simulink model "Arduino_model"  (R2021a)
settings: Solver=FixedStepAuto  StartTime=0.0  StopTime=inf  FixedStep=0.01  RelTol=1e-3  EnableMultiTasking=on
libraries: arduinolib x4, pid_lib x1, dspsigops x1, svdutilitieslib x1
settings Model: SimulationMode=external  SILPILModeSetting=veronly  ExtModeTrigDuration=2  Creator=s269684  LastModifiedBy=root
settings OptimizationCC: EnhancedBackFolding=on  PassReuseOutputArgsAs=Individual arguments  ZeroExternalMemoryAtStartup=off  ZeroInternalMemoryAtStartup=off  MaxStackSize=64  OptimizeBlockOrder=speed  DifferentSizesBufferReuse=on  OptimizationCustomize=off  EfficientTunableParamExpr=on
settings DebuggingCC: ParameterTunabilityLossMsg=error
settings HardwareCC: ProdBitPerInt=16  ProdBitPerPointer=16  ProdBitPerSizeT=16  ProdBitPerPtrDiffT=16  ProdLargestAtomicFloat=None  ProdWordSize=8  ProdHWDeviceType=Atmel->AVR  UseEmbeddedCoderFeatures=off
settings SFSimCC: MATLABDynamicMemAlloc=off
settings RTWCC: SystemTargetFile=ert.tlc  HardwareBoard=Arduino Uno  TemplateMakefile=ert_default_tmf  Toolchain=Arduino AVR  BuildConfiguration=Faster Runs
settings CodeAppCC: ForceParamTrailComments=on  IgnoreCustomStorageClasses=off  OperatorAnnotations=on  SimulinkDataObjDesc=on  SFDataObjDesc=on  InsertBlockDesc=on
settings ERTTargetCC: SupportContinuousTime=on  SupportNonInlinedSFcns=on  SupportVariableSizeSignals=on  ExtModeStaticAllocSize=250

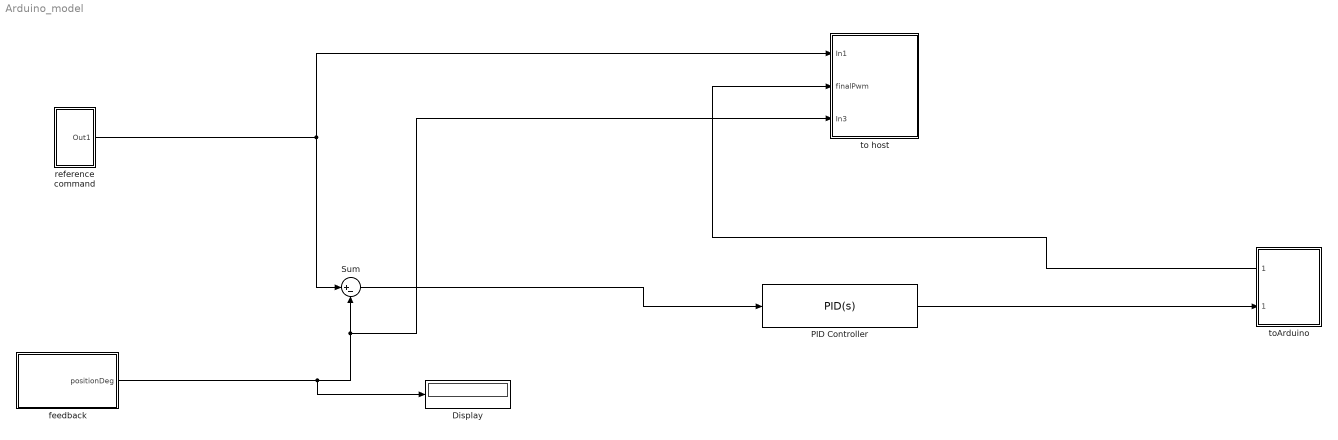
== system Arduino_model ==
  Display : Display
  PID Controller : pid_lib/PID Controller  Controller=PID  Form=Parallel  TimeDomain=Continuous-time  UseExternalTs=off  SampleTime=-1  IntegratorMethod=Forward Euler  FilterMethod=Forward Euler  ControllerParametersSource=internal  P=0.1  I=0  D=0  UseFilter=on  N=100  TunerSelectOption=Transfer Function Based (PID Tuner App)  InitialConditionSource=internal  InitialConditionForIntegrator=0  InitialConditionForFilter=0  DifferentiatorICPrevScaledInput=0  ExternalReset=none  TrackingMode=off  Kt=1  LimitOutput=off  SatLimitsSource=internal  UpperSaturationLimit=inf  LowerSaturationLimit=-inf  LinearizeAsGain=on  AntiWindupMode=none  Kb=1  POutMin=[]  POutMax=[]  IOutMin=[]  IOutMax=[]  DOutMin=[]  DOutMax=[]  NOutMin=[]  NOutMax=[]  SumOutMin=[]  SumOutMax=[]  SaturationOutMin=[]  SaturationOutMax=[]  PParamMin=[]  PParamMax=[]  IParamMin=[]  IParamMax=[]  DParamMin=[]  DParamMax=[]  NParamMin=[]  NParamMax=[]  KbParamMin=[]  KbParamMax=[]  KtParamMin=[]  KtParamMax=[]  KbOutMin=[]  KbOutMax=[]  KtOutMin=[]  KtOutMax=[]  IntegratorOutMin=[]  IntegratorOutMax=[]  FilterOutMin=[]  FilterOutMax=[]  SumI1OutMin=[]  SumI1OutMax=[]  SumI2OutMin=[]  SumI2OutMax=[]  SumI3OutMin=[]  SumI3OutMax=[]  SumI4OutMin=[]  SumI4OutMax=[]  SumDOutMin=[]  SumDOutMax=[]  DifferentiatorOutMin=[]  DifferentiatorOutMax=[]  FilterDiffOutCoefMin=[]  FilterDiffOutCoefMax=[]  ReciprocalOutMin=[]  ReciprocalOutMax=[]  SumDenOutMin=[]  SumDenOutMax=[]  SumNumOutMin=[]  SumNumOutMax=[]  DivideOutMin=[]  DivideOutMax=[]  UdiffTsProdOutMin=[]  UdiffTsProdOutMax=[]  NTsProdOutMin=[]  NTsProdOutMax=[]  UintegralTsProdOutMin=[]  UintegralTsProdOutMax=[]  UngainTsProdOutMin=[]  UngainTsProdOutMax=[]  IntegratorContinuousStateAttributes=''  IntegratorStateMustResolveToSignalObject=off  IntegratorRTWStateStorageClass=Auto  FilterContinuousStateAttributes=''  FilterStateMustResolveToSignalObject=off  FilterRTWStateStorageClass=Auto  ParallelPVariant=InternalParameters  IdealPVariant=Disabled  IVariant=InternalParameters  DVariant=InternalParameters  IntegratorVariant=Continuous  SatVariant=Disabled  AWVariant=Passthrough  PCopyVariant=Disabled  TRVariant=Disabled  FdbkBlocksVariant=Forward  IdealPFdbkVariant=Disabled  SatFdbkVariant=Disabled  DerivativeFilterVariant=ContFilter  NVariant=InternalParameters  NCopyVariant=Disabled  FilterICVariant=InternalICsFilter  IntegratorICVariant=InternalICs  ExternalResetVariant=Disabled  TRSumVariant=Passthrough  SumFdbkVariant=Disabled  SumVariant=Sum_PID  TsampFilterVariant=InternalTs  TsampNgainVariant=Passthrough  TsampIntegralVariant=Passthrough  ExternalSaturationOutDataTypeStr=Inherit: Same as second input
  Sum : Sum  Inputs=|+-
  feedback : Subsystem
  reference command : Subsystem
  to host : Subsystem
  toArduino : Subsystem
      settings: PortSchema="{\"entries\":[{\"content\":{\"sides\":[{\"content\":{\"connectorIds\":[\"Out1\",\"In1\"]},\"type\":\"ConnectorPlacement.EquallySpacedRectSide\",\"uuid\":\"00d106dc-c9fd-4c71-abfc-8846c8674c7f\"},{\"content\":{\"connectorIds\":[],\"side\":\"RIGHT\"},\"type\":\"ConnectorPlacement.EquallySpacedRectSide\",\"uuid\":\"650a5093-1d9f-4912-81bc-53c75c5aa512\"},{\"content\":{\"connectorIds\":[],\"side\":\"TOP\"},\"type\":\"ConnectorPlacement.EquallySpacedRectSide\",\"uuid\":\"91886ec9-88b3-4850-970c-16eb2204124f\"}]},\"type\":\"ConnectorPlacement.EquallySpacedConnector\",\"uuid\":\"6b0efc47-7dc5-4517-b0e2-3344f600596a\"}],\"packageUris\":[\"http://schema.mathworks.com/mf0/Connector/R2020b\"],\"version\":\"1.0\"}"
  wires:
  feedback/1(positionDeg) -> Display/1, to host/3(In3), Sum/2
  Sum/1 -> PID Controller/1
  PID Controller/1 -> toArduino/1(motorTrq)
  toArduino/1(finalPwm) -> to host/2(finalPwm)
  reference command/1(Out1) -> Sum/1, to host/1(In1)

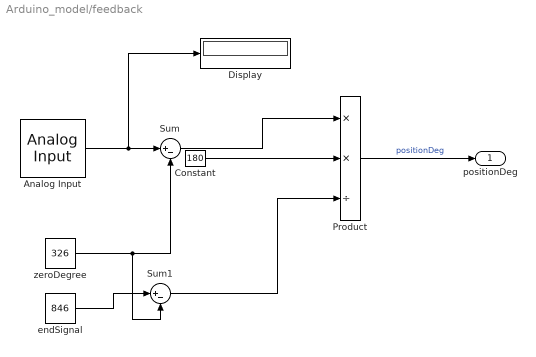
== system Arduino_model/feedback ==
  Analog Input : arduinolib/Analog Input  pinNumber=1  ReadResultsOnly=off  ConversionTriggerSource=Software  ExternalTriggerType=uint32( 0 )  OutputDataType=uint16  EnableConversionCompleteNotify=off  EnableOuputStatus=off  SampleTime=-1  blockPlatform=arduino
  Constant : Constant  Value=180
  Display : Display
  Product : Product  Inputs=**/
  Sum : Sum  Inputs=|+-
  Sum1 : Sum  Inputs=|+-
  endSignal : Constant  Value=846
  zeroDegree : Constant  Value=326
  positionDeg : Outport
  wires:
  Sum/1 -> Product/1
  Product/1 -> positionDeg/1  "positionDeg"
  Constant/1 -> Product/2
  zeroDegree/1 -> Sum/2, Sum1/2
  Sum1/1 -> Product/3
  Analog Input/1 -> Display/1, Sum/1
  endSignal/1 -> Sum1/1

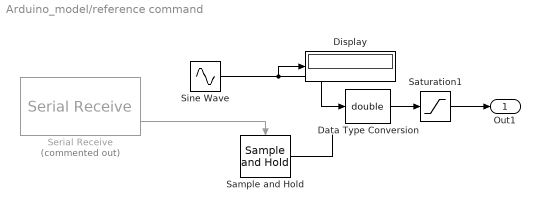
== system Arduino_model/reference command ==
  Data Type Conversion : DataTypeConversion  OutDataTypeStr=double
  Display : Display
  Sample and Hold : dspsigops/Sample and Hold  trig=Rising edge  initCond=0  latchinput=off
  Saturation1 : Saturate  UpperLimit=165  LowerLimit=20
  Serial Receive : arduinolib/Serial Receive  Commented=on  isARMArch=off  portNumber=0  DataType=uint8  Datalength=1  SampleTime=0.01  showOutStatus=on  blockPlatform=arduino
      settings: SourceProductBaseCode=ARDUINO
  Sine Wave : Sin  Amplitude=45  Bias=90  Frequency=10  SampleTime=0
  Out1 : Outport
  wires:
  Data Type Conversion/1 -> Saturation1/1
  Serial Receive/2 -> Sample and Hold/Trigger
  Sine Wave/1 -> Display/1, Data Type Conversion/1
  Saturation1/1 -> Out1/1
  Sample and Hold/1 -> ?

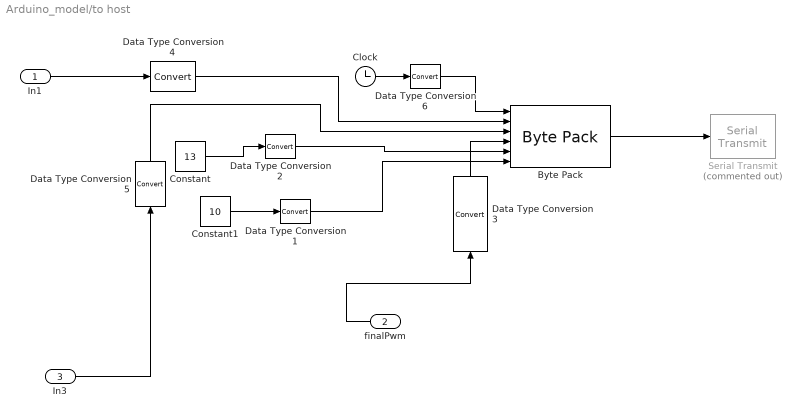
== system Arduino_model/to host ==
  In1 : Inport
  finalPwm : Inport  Port=2
  In3 : Inport  Port=3
  Byte Pack : svdutilitieslib/Byte Pack  maskPackedDataType=uint8  datatypes={'single' , 'single', 'single', 'single', 'uint8', 'uint8'}  byteAlign=1  blockPlatform=arduinoert
      settings: SourceProductBaseCode=ANDROID,ARDUINO,ML_ARDUINO,ECCORTEXA,ECCORTEXR,SC_BEAGLEBONE_BLUE,EC_FREEDOM_BOARD,EC_FRDM_K64F,INTEL_BLOCKSET,JETSONCPU,MICROBIT,NUCLEO,NVIDIA,PX4AUTOPILOTS,RASPPIIO,STMICRODIS,TIC2000,XILINX_BLOCKSET
  Clock : Clock
  Constant : Constant  Value=13
  Constant1 : Constant  Value=10
  Data Type Conversion{1..6} (6 alike) : DataTypeConversion
  Serial Transmit : arduinolib/Serial Transmit  Commented=on  portNumber=0  sendmode=write  sendformat=Decimal  floatprecision=2  blockPlatform=arduino
  wires:
  finalPwm/1 -> Data Type Conversion3/1
  Data Type Conversion5/1 -> Byte Pack/3
  Data Type Conversion4/1 -> Byte Pack/2
  Data Type Conversion1/1 -> Byte Pack/6
  Constant/1 -> Data Type Conversion2/1
  Constant1/1 -> Data Type Conversion1/1
  Data Type Conversion2/1 -> Byte Pack/5
  Byte Pack/1 -> Serial Transmit/1
  In3/1 -> Data Type Conversion5/1
  In1/1 -> Data Type Conversion4/1
  Data Type Conversion3/1 -> Byte Pack/4
  Clock/1 -> Data Type Conversion6/1
  Data Type Conversion6/1 -> Byte Pack/1

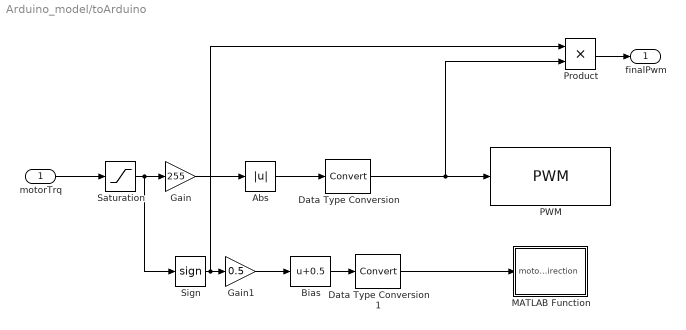
== system Arduino_model/toArduino ==
  motorTrq : Inport
  Abs : Abs
  Bias : Bias  Bias=0.5
  Data Type Conversion : DataTypeConversion
  Data Type Conversion1 : DataTypeConversion
  Gain : Gain  Gain=255
  Gain1 : Gain  Gain=0.5
  MATLAB Function : MATLAB Function  TreatAsAtomicUnit=on
  PWM : arduinolib/PWM  pinNumber=6  frequencyType=Default  desiredFrequency=490.2  achievableFrequency=490.2
  Product : Product
  Saturation : Saturate  UpperLimit=1  LowerLimit=-1
  Sign : Signum
  finalPwm : Outport
  wires:
  Data Type Conversion/1 -> Product/2, PWM/1
  motorTrq/1 -> Saturation/1
  Saturation/1 -> Sign/1, Gain/1
  Gain/1 -> Abs/1
  Sign/1 -> Product/1, Gain1/1
  Gain1/1 -> Bias/1
  Bias/1 -> Data Type Conversion1/1
  Data Type Conversion1/1 -> MATLAB Function/1(motorDirection)
  Abs/1 -> Data Type Conversion/1
  Product/1 -> finalPwm/1

== matlab function Arduino_model/toArduino/MATLAB Function ==
  data: motorDirection input
function fcn(motorDirection)
persistent arduinoObj;
directionPin = "A0";
if (isempty(arduinoObj))
    arduinoObj = arduino();
    arduinoObj.configurePin(directionPin , "DigitalOutput");
end

arduinoObj.writeDigitalPin(directionPin, motorDirection)
end
